simulink model "sheet"  (R2021b)
settings: Solver=VariableStepAuto  StartTime=0.0  StopTime=1.0  RelTol=1e-3
undefined symbols (not defined in the file): den, gain, init, num
settings Model: Creator=Саня  LastModifiedBy=roman

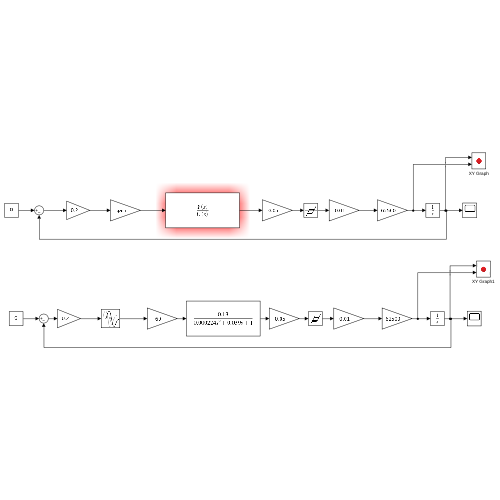
[thumbnail: Simulink's stored preview of the top-level diagram]
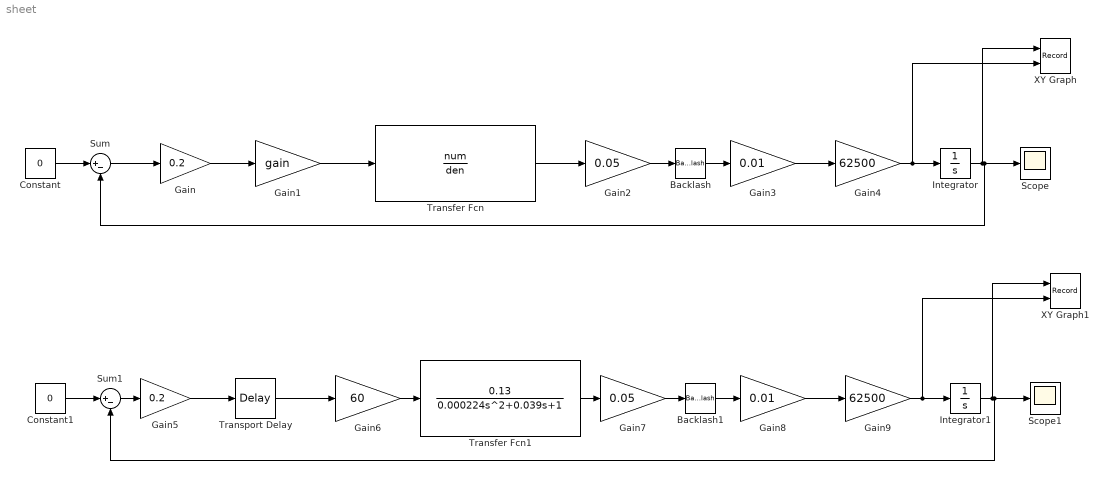
== system sheet ==
  Backlash : Backlash  BacklashWidth=1e-6
  Backlash1 : Backlash  BacklashWidth=1e-6
  Constant : Constant  Value=0
  Constant1 : Constant  Value=0
  Gain : Gain  Gain=0.2
  Gain1 : Gain  Gain=gain
  Gain2 : Gain  Gain=0.05
  Gain3 : Gain  Gain=0.01
  Gain4 : Gain  Gain=62500
  Gain5 : Gain  Gain=0.2
  Gain6 : Gain  Gain=60
  Gain7 : Gain  Gain=0.05
  Gain8 : Gain  Gain=0.01
  Gain9 : Gain  Gain=62500
  Integrator : Integrator  InitialCondition=init
  Integrator1 : Integrator  InitialCondition=12800
  Scope : Scope
  Scope1 : Scope
  Sum : Sum  Inputs=|+-
  Sum1 : Sum  Inputs=|+-
  Transfer Fcn : TransferFcn  Numerator=num  Denominator=den
  Transfer Fcn1 : TransferFcn  Numerator=[0.13]  Denominator=[0.000224 0.039 1]
  Transport Delay : TransportDelay  DelayTime=0.007
  XY Graph : Record  FileSettingsInternal="{\"entries\":[{\"content\":{\"excelSettings\":{\"content\":{},\"type\":\"Streamout.ExcelSettings\"}},\"type\":\"Streamout.FileSettingStorage\",\"uuid\":\"939fa1e9-9014-4588-975e-be3bc9622890\"}],\"packageUris\":[\"http://schema.mathworks.com/mf0/streamout_blocks/R2020a\"],\"version\":\"1.0\"}"  Layout=[1 1]  SignalsInternal="{\"entries\":[{\"content\":{\"signals\":[{\"content\":{\"blockPath\":[\"sheet/XY Graph\"],\"channel\":[],\"dimensions\":[1],\"domain\":\"sheet/XY Graph\",\"lineColor\":\"#a2142f\",\"plots\":[1],\"port\":1,\"sid\":[\"\"],\"signalID\":148,\"signalName\":\"Integrator\"},\"type\":\"RecordBlkView.Signal\",\"uuid\":\"c185cff9-2223-4105-a9d3-27881c75aa36\"},{\"content\":{\"blockPath\":[\"sheet/XY Graph\"],\"channel\":[],\"dimensions\":[1],\"domain\":\"sheet/XY Graph\",\"lineColor\":\"#139fff\",\"plots\":[1],\"port\":2,\"sid\":[\"\"],\"signalID\":152,\"signalName\":\"Gain4\"},\"type\":\"RecordBlkView.Signal\",\"uuid\":\"db002b79-c8c9-4033-ae17-6fd173603baf\"}]},\"type\":\"RecordBlkView.InputSignals\",\"uuid\":\"38fe68d5-25c0-4729-8ce5-c9dc347f7c42\"}],\"packageUris\":[\"http://schema.mathworks.com/mf0/streamout_blocks/R2020a\"],\"version\":\"1.0\"}"  VisualizationBindings="{\"xyplotplugin\":{\"info\":[{\"series\":[{\"bindingParametersList\":[{\"parameter\":\"X-Axis\",\"signalID\":148,\"signalName\":\"Integrator\"},{\"parameter\":\"Y-Axis\",\"signalID\":152,\"signalName\":\"Gain4\"}],\"seriesID\":54820}],\"subplotID\":1}]}}"  CompatibilityTag=XY  st=-1
  XY Graph1 : Record  FileSettingsInternal="{\"entries\":[{\"content\":{\"excelSettings\":{\"content\":{},\"type\":\"Streamout.ExcelSettings\"}},\"type\":\"Streamout.FileSettingStorage\",\"uuid\":\"89391693-272d-48b6-9504-7290b2afa889\"}],\"packageUris\":[\"http://schema.mathworks.com/mf0/streamout_blocks/R2020a\"],\"version\":\"1.0\"}"  Layout=[1 1]  SignalsInternal="{\"entries\":[{\"content\":{\"signals\":[{\"content\":{\"blockPath\":[\"sheet/XY Graph1\"],\"channel\":[],\"dimensions\":[1],\"domain\":\"sheet/XY Graph1\",\"lineColor\":\"#a2142f\",\"plots\":[1],\"port\":1,\"sid\":[\"\"],\"signalID\":156,\"signalName\":\"Integrator1\"},\"type\":\"RecordBlkView.Signal\",\"uuid\":\"0cfce138-2e20-4626-8340-9aee0e6c6cae\"},{\"content\":{\"blockPath\":[\"sheet/XY Graph1\"],\"channel\":[],\"dimensions\":[1],\"domain\":\"sheet/XY Graph1\",\"lineColor\":\"#139fff\",\"plots\":[1],\"port\":2,\"sid\":[\"\"],\"signalID\":160,\"signalName\":\"Gain9\"},\"type\":\"RecordBlkView.Signal\",\"uuid\":\"446c3f78-31c3-491b-bb92-38504dc8f772\"}]},\"type\":\"RecordBlkView.InputSignals\",\"uuid\":\"5e71d692-f8b9-4ecc-9cda-e4aec156ffa3\"}],\"packageUris\":[\"http://schema.mathworks.com/mf0/streamout_blocks/R2020a\"],\"version\":\"1.0\"}"  VisualizationBindings="{\"xyplotplugin\":{\"info\":[{\"series\":[{\"bindingParametersList\":[{\"parameter\":\"X-Axis\",\"signalID\":156,\"signalName\":\"Integrator1\"},{\"parameter\":\"Y-Axis\",\"signalID\":160,\"signalName\":\"Gain9\"}],\"seriesID\":44728}],\"subplotID\":1}]}}"  CompatibilityTag=XY  st=-1
  wires:
  Constant/1 -> Sum/1
  Sum/1 -> Gain/1
  Gain/1 -> Gain1/1
  Gain1/1 -> Transfer Fcn/1
  Transfer Fcn/1 -> Gain2/1
  Gain2/1 -> Backlash/1
  Backlash/1 -> Gain3/1
  Gain3/1 -> Gain4/1
  Gain4/1 -> XY Graph/2, Integrator/1
  Integrator/1 -> XY Graph/1, Sum/2, Scope/1
  Gain7/1 -> Backlash1/1
  Transfer Fcn1/1 -> Gain7/1
  Gain6/1 -> Transfer Fcn1/1
  Backlash1/1 -> Gain8/1
  Sum1/1 -> Gain5/1
  Constant1/1 -> Sum1/1
  Integrator1/1 -> XY Graph1/1, Sum1/2, Scope1/1
  Gain9/1 -> XY Graph1/2, Integrator1/1
  Gain8/1 -> Gain9/1
  Transport Delay/1 -> Gain6/1
  Gain5/1 -> Transport Delay/1
